simulink model "MATE_PMSMDynamicSwitches"  (R2024b)
settings: Solver=FixedStepDiscrete  StartTime=0.0  StopTime=0.6  RelTol=1e-3  AbsTol=1e-3
PostLoadFcn:
  | Ts = 2e-6;
  | PMSMDynamicSwitches_init
InitFcn:
  | Ts = 2e-6;
  | PMSMDynamicSwitches_init
values from neighbouring files (symbols this model uses):
  J = 0.2    [PMSMDynamicSwitches_init.m]
  Tmax = 1.5*N*PM*Imax    (= 27)    [PMSMDynamicSwitches_init.m]
  Tsc = 1/fc    (= 5e-05)    [PMSMDynamicSwitches_init.m]
libraries: fl_lib x24, nesl_utility x19, simulink x3, ee_lib x3, batteryecm_lib x1, eePmsmFieldOrientedControl x1
(part 2 of 2)

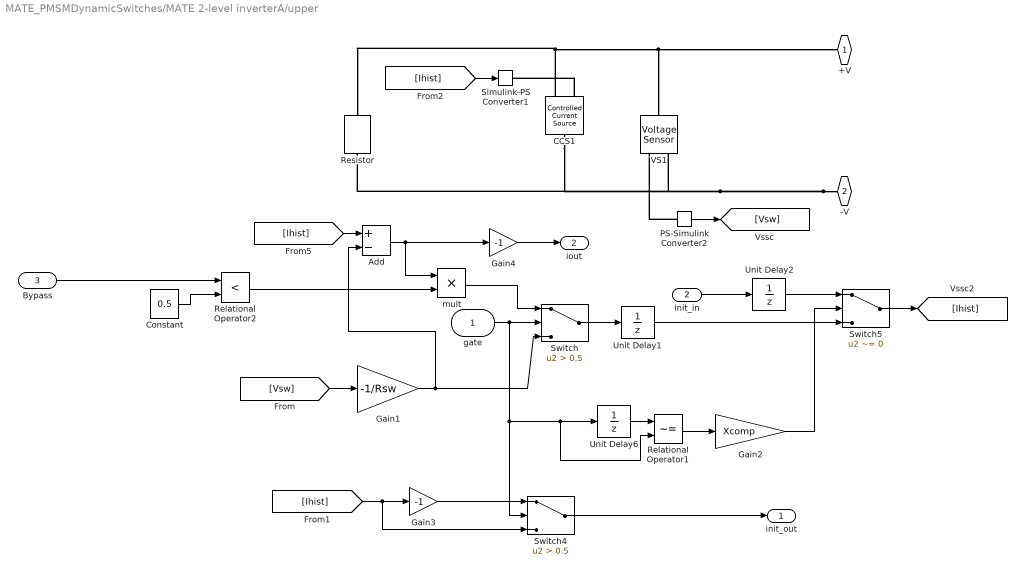
== system MATE_PMSMDynamicSwitches/MATE 2-level inverterA/upper ==
  gate : Inport
  init_in : Inport  Port=2
  Bypass : Inport  Port=3
  Add : Sum  Inputs=+-
  CCS1 : fl_lib/Electrical/Electrical Sources/Controlled Current Source
  Constant : Constant  Value=0.5
  Gain1 : Gain  Gain=-1/Rsw
  Gain2 : Gain  Gain=Xcomp
  Gain3 : Gain  Gain=-1
  Gain4 : Gain  Gain=-1
  PS-Simulink Converter2 : nesl_utility/PS-Simulink Converter  PhysicalDomain=network_engine_domain  SubClassName=ps_output  LeftPortType=input  RightPortType=output  PseudoPeriodic=off  Frequencies=[]  VectorFormat=inherit  Unit=inherit  AffineConversion=off
  Relational Operator1 : RelationalOperator  Operator=~=  OutDataTypeStr=boolean  RndMeth=Simplest  InputSameDT=off
  Relational Operator2 : RelationalOperator  Operator=<  OutDataTypeStr=boolean  RndMeth=Simplest  InputSameDT=off
  Resistor : fl_lib/Electrical/Electrical Elements/Resistor  R=Rsw Ohm  i_specify=off  i_priority=None  i=0 A  i_nominal_specify=off  i_nominal_value=1  i_nominal_unit=A  v_specify=off  v_priority=None  v=0 V  v_nominal_specify=off  v_nominal_value=1  v_nominal_unit=V
  Simulink-PS Converter1 : nesl_utility/Simulink-PS Converter  PhysicalDomain=network_engine_domain  SubClassName=ps_input  LeftPortType=input  RightPortType=output  PseudoPeriodic=off  Frequencies=[]  NoiseDistribution=none  NoiseParameters=[]  Unit=1  AffineConversion=off  FilteringAndDerivatives=provide  SimscapeFilterOrder=1  InputFilterTimeConstant=0.001  UdotUserProvided=0
  Switch : Switch  Criteria=u2 > Threshold  Threshold=0.5  SaturateOnIntegerOverflow=off  InputSameDT=off
  Switch4 : Switch  Criteria=u2 > Threshold  Threshold=0.5  SaturateOnIntegerOverflow=off  InputSameDT=off
  Switch5 : Switch  Criteria=u2 ~= 0  Threshold=0.5  SaturateOnIntegerOverflow=off  InputSameDT=off
  Unit Delay1 : UnitDelay  SampleTime=-1  HasFrameUpgradeWarning=on
  Unit Delay2 : UnitDelay  SampleTime=Ts  HasFrameUpgradeWarning=on
  Unit Delay6 : UnitDelay  SampleTime=Ts  HasFrameUpgradeWarning=on
  VS1 : fl_lib/Electrical/Electrical Sensors/Voltage Sensor
  mult : Product
  +V : PMIOPort  Side=Left
  -V : PMIOPort  Port=2  Side=Right
  init_out : Outport
  iout : Outport  Port=2
  wires:
  Constant/1 -> Relational Operator2/2
  Unit Delay2/1 -> Switch5/1
  [Ihist] -> Gain3/1, Switch4/3
  Relational Operator2/1 -> mult/2
  Bypass/1 -> Relational Operator2/1
  mult/1 -> Switch/1
  [Ihist] -> Simulink-PS Converter1/1
  Switch/1 -> Unit Delay1/1
  [Vsw] -> Gain1/1
  PS-Simulink Converter2/1 -> [Vsw]
  [Ihist] -> Add/1
  Gain1/1 -> Switch/3, Add/2
  Add/1 -> Gain4/1, mult/1
  Unit Delay1/1 -> Switch5/3
  Switch4/1 -> init_out/1
  Gain3/1 -> Switch4/1
  Gain2/1 -> Switch5/2
  Unit Delay6/1 -> Relational Operator1/1
  gate/1 -> Switch4/2, Unit Delay6/1, Relational Operator1/2, Switch/2
  Relational Operator1/1 -> Gain2/1
  init_in/1 -> Unit Delay2/1
  Switch5/1 -> [Ihist]
  Gain4/1 -> iout/1
  connections:
  CCS1/RConn2 -- +V/RConn1 -- VS1/LConn1 -- Resistor/LConn1
  CCS1/RConn1 -- Simulink-PS Converter1/RConn1
  PS-Simulink Converter2/LConn1 -- VS1/RConn1
  -V/RConn1 -- VS1/RConn2 -- CCS1/LConn1 -- Resistor/RConn1

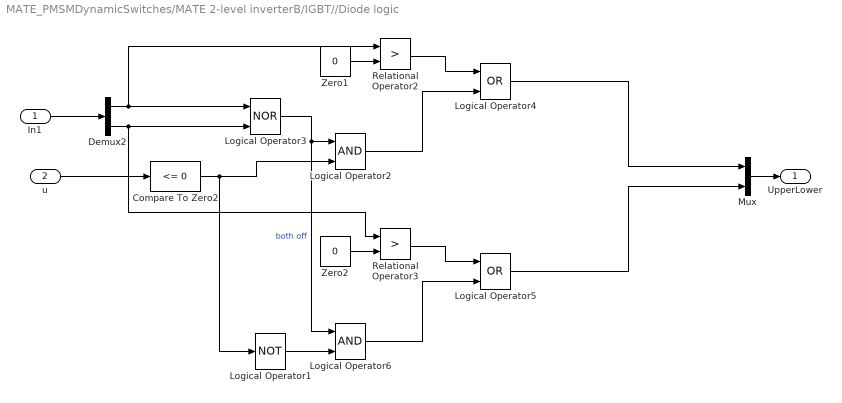
== system MATE_PMSMDynamicSwitches/MATE 2-level inverterB/IGBT//Diode logic ==
  In1 : Inport
  u : Inport  Port=2
  Compare To Zero2 : simulink/Logic and Bit Operations/Compare To Zero  relop=<=  OutDataTypeStr=uint8
  Demux2 : Demux  Outputs=2
  Logical Operator1 : Logic  Operator=NOT  AllPortsSameDT=off  OutDataTypeStr=boolean
  Logical Operator2 : Logic  AllPortsSameDT=off  OutDataTypeStr=boolean
  Logical Operator3 : Logic  Operator=NOR  AllPortsSameDT=off  OutDataTypeStr=boolean
  Logical Operator4 : Logic  Operator=OR  AllPortsSameDT=off  OutDataTypeStr=boolean
  Logical Operator5 : Logic  Operator=OR  AllPortsSameDT=off  OutDataTypeStr=boolean
  Logical Operator6 : Logic  AllPortsSameDT=off  OutDataTypeStr=boolean
  Mux : Mux  Inputs=2
  Relational Operator2 : RelationalOperator  Operator=>  OutDataTypeStr=boolean  InputSameDT=off
  Relational Operator3 : RelationalOperator  Operator=>  OutDataTypeStr=boolean  InputSameDT=off
  Zero1 : Constant  Value=0  OutDataTypeStr=Inherit: Inherit via back propagation
  Zero2 : Constant  Value=0  OutDataTypeStr=Inherit: Inherit via back propagation
  UpperLower : Outport
  wires:
  Mux/1 -> UpperLower/1
  Logical Operator5/1 -> Mux/2
  Logical Operator4/1 -> Mux/1
  In1/1 -> Demux2/1
  u/1 -> Compare To Zero2/1
  Logical Operator1/1 -> Logical Operator6/2
  Relational Operator3/1 -> Logical Operator5/1
  Logical Operator2/1 -> Logical Operator4/2
  Zero2/1 -> Relational Operator3/2
  Demux2/2 -> Relational Operator3/1, Logical Operator3/2
  Logical Operator6/1 -> Logical Operator5/2
  Compare To Zero2/1 -> Logical Operator2/2, Logical Operator1/1
  Zero1/1 -> Relational Operator2/2
  Logical Operator3/1 -> Logical Operator2/1, Logical Operator6/1  "both off"
  Relational Operator2/1 -> Logical Operator4/1
  Demux2/1 -> Relational Operator2/1, Logical Operator3/1

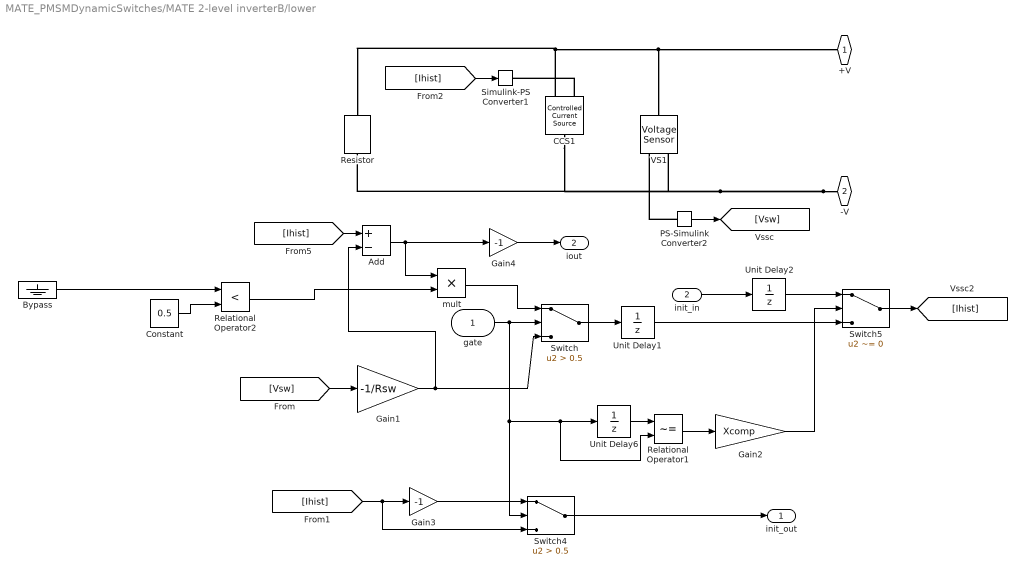
== system MATE_PMSMDynamicSwitches/MATE 2-level inverterB/lower ==
  gate : Inport
  init_in : Inport  Port=2
  Add : Sum  Inputs=+-
  Bypass : Ground
  CCS1 : fl_lib/Electrical/Electrical Sources/Controlled Current Source
  Constant : Constant  Value=0.5
  Gain1 : Gain  Gain=-1/Rsw
  Gain2 : Gain  Gain=Xcomp
  Gain3 : Gain  Gain=-1
  Gain4 : Gain  Gain=-1
  PS-Simulink Converter2 : nesl_utility/PS-Simulink Converter  PhysicalDomain=network_engine_domain  SubClassName=ps_output  LeftPortType=input  RightPortType=output  PseudoPeriodic=off  Frequencies=[]  VectorFormat=inherit  Unit=inherit  AffineConversion=off
  Relational Operator1 : RelationalOperator  Operator=~=  OutDataTypeStr=boolean  RndMeth=Simplest  InputSameDT=off
  Relational Operator2 : RelationalOperator  Operator=<  OutDataTypeStr=boolean  RndMeth=Simplest  InputSameDT=off
  Resistor : fl_lib/Electrical/Electrical Elements/Resistor  R=Rsw Ohm  i_specify=off  i_priority=None  i=0 A  i_nominal_specify=off  i_nominal_value=1  i_nominal_unit=A  v_specify=off  v_priority=None  v=0 V  v_nominal_specify=off  v_nominal_value=1  v_nominal_unit=V
  Simulink-PS Converter1 : nesl_utility/Simulink-PS Converter  PhysicalDomain=network_engine_domain  SubClassName=ps_input  LeftPortType=input  RightPortType=output  PseudoPeriodic=off  Frequencies=[]  NoiseDistribution=none  NoiseParameters=[]  Unit=1  AffineConversion=off  FilteringAndDerivatives=provide  SimscapeFilterOrder=1  InputFilterTimeConstant=0.001  UdotUserProvided=0
  Switch : Switch  Criteria=u2 > Threshold  Threshold=0.5  SaturateOnIntegerOverflow=off  InputSameDT=off
  Switch4 : Switch  Criteria=u2 > Threshold  Threshold=0.5  SaturateOnIntegerOverflow=off  InputSameDT=off
  Switch5 : Switch  Criteria=u2 ~= 0  Threshold=0.5  SaturateOnIntegerOverflow=off  InputSameDT=off
  Unit Delay1 : UnitDelay  SampleTime=-1  HasFrameUpgradeWarning=on
  Unit Delay2 : UnitDelay  SampleTime=Ts  HasFrameUpgradeWarning=on
  Unit Delay6 : UnitDelay  SampleTime=Ts  HasFrameUpgradeWarning=on
  VS1 : fl_lib/Electrical/Electrical Sensors/Voltage Sensor
  mult : Product
  +V : PMIOPort  Side=Left
  -V : PMIOPort  Port=2  Side=Right
  init_out : Outport
  iout : Outport  Port=2
  wires:
  Constant/1 -> Relational Operator2/2
  Unit Delay2/1 -> Switch5/1
  [Ihist] -> Gain3/1, Switch4/3
  Relational Operator2/1 -> mult/2
  Bypass/1 -> Relational Operator2/1
  mult/1 -> Switch/1
  [Ihist] -> Simulink-PS Converter1/1
  Switch/1 -> Unit Delay1/1
  [Vsw] -> Gain1/1
  PS-Simulink Converter2/1 -> [Vsw]
  [Ihist] -> Add/1
  Gain1/1 -> Switch/3, Add/2
  Add/1 -> Gain4/1, mult/1
  Unit Delay1/1 -> Switch5/3
  Switch4/1 -> init_out/1
  Gain3/1 -> Switch4/1
  Gain2/1 -> Switch5/2
  Unit Delay6/1 -> Relational Operator1/1
  gate/1 -> Switch4/2, Unit Delay6/1, Relational Operator1/2, Switch/2
  Relational Operator1/1 -> Gain2/1
  init_in/1 -> Unit Delay2/1
  Switch5/1 -> [Ihist]
  Gain4/1 -> iout/1
  connections:
  CCS1/RConn2 -- +V/RConn1 -- VS1/LConn1 -- Resistor/LConn1
  CCS1/RConn1 -- Simulink-PS Converter1/RConn1
  PS-Simulink Converter2/LConn1 -- VS1/RConn1
  -V/RConn1 -- VS1/RConn2 -- CCS1/LConn1 -- Resistor/RConn1

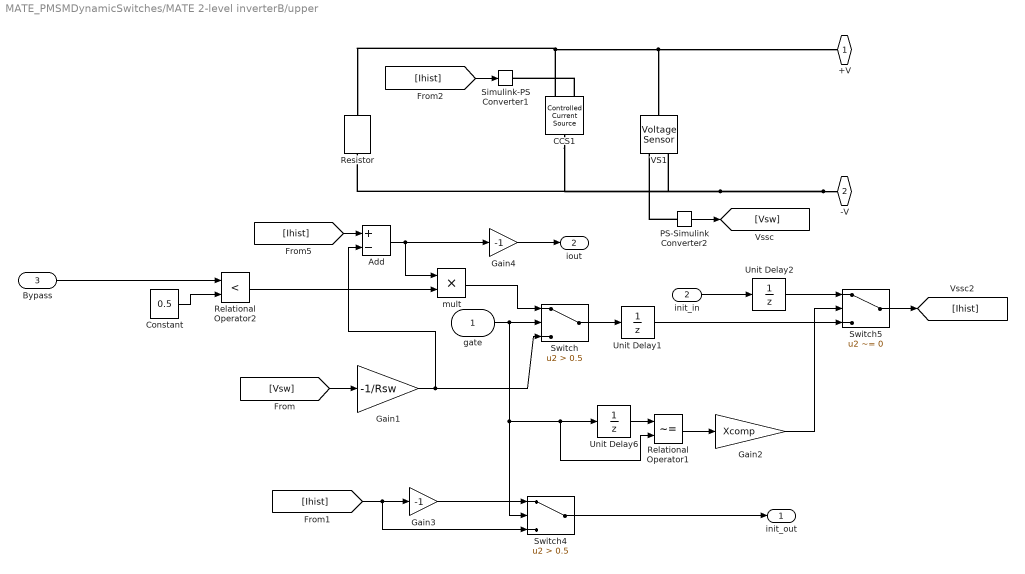
== system MATE_PMSMDynamicSwitches/MATE 2-level inverterB/upper ==
  gate : Inport
  init_in : Inport  Port=2
  Bypass : Inport  Port=3
  Add : Sum  Inputs=+-
  CCS1 : fl_lib/Electrical/Electrical Sources/Controlled Current Source
  Constant : Constant  Value=0.5
  Gain1 : Gain  Gain=-1/Rsw
  Gain2 : Gain  Gain=Xcomp
  Gain3 : Gain  Gain=-1
  Gain4 : Gain  Gain=-1
  PS-Simulink Converter2 : nesl_utility/PS-Simulink Converter  PhysicalDomain=network_engine_domain  SubClassName=ps_output  LeftPortType=input  RightPortType=output  PseudoPeriodic=off  Frequencies=[]  VectorFormat=inherit  Unit=inherit  AffineConversion=off
  Relational Operator1 : RelationalOperator  Operator=~=  OutDataTypeStr=boolean  RndMeth=Simplest  InputSameDT=off
  Relational Operator2 : RelationalOperator  Operator=<  OutDataTypeStr=boolean  RndMeth=Simplest  InputSameDT=off
  Resistor : fl_lib/Electrical/Electrical Elements/Resistor  R=Rsw Ohm  i_specify=off  i_priority=None  i=0 A  i_nominal_specify=off  i_nominal_value=1  i_nominal_unit=A  v_specify=off  v_priority=None  v=0 V  v_nominal_specify=off  v_nominal_value=1  v_nominal_unit=V
  Simulink-PS Converter1 : nesl_utility/Simulink-PS Converter  PhysicalDomain=network_engine_domain  SubClassName=ps_input  LeftPortType=input  RightPortType=output  PseudoPeriodic=off  Frequencies=[]  NoiseDistribution=none  NoiseParameters=[]  Unit=1  AffineConversion=off  FilteringAndDerivatives=provide  SimscapeFilterOrder=1  InputFilterTimeConstant=0.001  UdotUserProvided=0
  Switch : Switch  Criteria=u2 > Threshold  Threshold=0.5  SaturateOnIntegerOverflow=off  InputSameDT=off
  Switch4 : Switch  Criteria=u2 > Threshold  Threshold=0.5  SaturateOnIntegerOverflow=off  InputSameDT=off
  Switch5 : Switch  Criteria=u2 ~= 0  Threshold=0.5  SaturateOnIntegerOverflow=off  InputSameDT=off
  Unit Delay1 : UnitDelay  SampleTime=-1  HasFrameUpgradeWarning=on
  Unit Delay2 : UnitDelay  SampleTime=Ts  HasFrameUpgradeWarning=on
  Unit Delay6 : UnitDelay  SampleTime=Ts  HasFrameUpgradeWarning=on
  VS1 : fl_lib/Electrical/Electrical Sensors/Voltage Sensor
  mult : Product
  +V : PMIOPort  Side=Left
  -V : PMIOPort  Port=2  Side=Right
  init_out : Outport
  iout : Outport  Port=2
  wires:
  Constant/1 -> Relational Operator2/2
  Unit Delay2/1 -> Switch5/1
  [Ihist] -> Gain3/1, Switch4/3
  Relational Operator2/1 -> mult/2
  Bypass/1 -> Relational Operator2/1
  mult/1 -> Switch/1
  [Ihist] -> Simulink-PS Converter1/1
  Switch/1 -> Unit Delay1/1
  [Vsw] -> Gain1/1
  PS-Simulink Converter2/1 -> [Vsw]
  [Ihist] -> Add/1
  Gain1/1 -> Switch/3, Add/2
  Add/1 -> Gain4/1, mult/1
  Unit Delay1/1 -> Switch5/3
  Switch4/1 -> init_out/1
  Gain3/1 -> Switch4/1
  Gain2/1 -> Switch5/2
  Unit Delay6/1 -> Relational Operator1/1
  gate/1 -> Switch4/2, Unit Delay6/1, Relational Operator1/2, Switch/2
  Relational Operator1/1 -> Gain2/1
  init_in/1 -> Unit Delay2/1
  Switch5/1 -> [Ihist]
  Gain4/1 -> iout/1
  connections:
  CCS1/RConn2 -- +V/RConn1 -- VS1/LConn1 -- Resistor/LConn1
  CCS1/RConn1 -- Simulink-PS Converter1/RConn1
  PS-Simulink Converter2/LConn1 -- VS1/RConn1
  -V/RConn1 -- VS1/RConn2 -- CCS1/LConn1 -- Resistor/RConn1

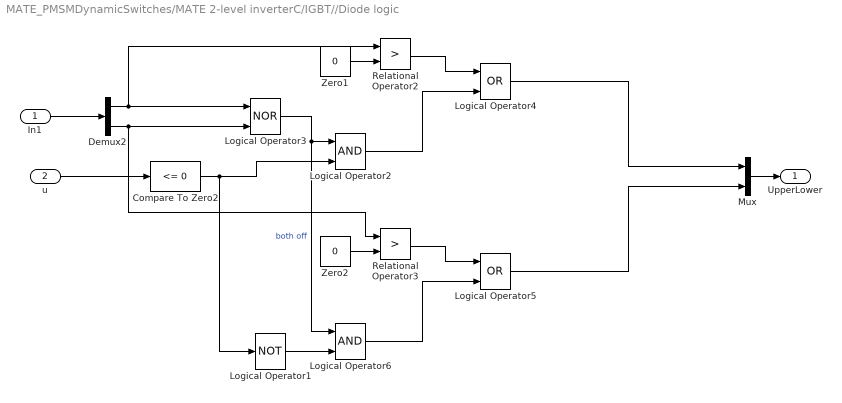
== system MATE_PMSMDynamicSwitches/MATE 2-level inverterC/IGBT//Diode logic ==
  In1 : Inport
  u : Inport  Port=2
  Compare To Zero2 : simulink/Logic and Bit Operations/Compare To Zero  relop=<=  OutDataTypeStr=uint8
  Demux2 : Demux  Outputs=2
  Logical Operator1 : Logic  Operator=NOT  AllPortsSameDT=off  OutDataTypeStr=boolean
  Logical Operator2 : Logic  AllPortsSameDT=off  OutDataTypeStr=boolean
  Logical Operator3 : Logic  Operator=NOR  AllPortsSameDT=off  OutDataTypeStr=boolean
  Logical Operator4 : Logic  Operator=OR  AllPortsSameDT=off  OutDataTypeStr=boolean
  Logical Operator5 : Logic  Operator=OR  AllPortsSameDT=off  OutDataTypeStr=boolean
  Logical Operator6 : Logic  AllPortsSameDT=off  OutDataTypeStr=boolean
  Mux : Mux  Inputs=2
  Relational Operator2 : RelationalOperator  Operator=>  OutDataTypeStr=boolean  InputSameDT=off
  Relational Operator3 : RelationalOperator  Operator=>  OutDataTypeStr=boolean  InputSameDT=off
  Zero1 : Constant  Value=0  OutDataTypeStr=Inherit: Inherit via back propagation
  Zero2 : Constant  Value=0  OutDataTypeStr=Inherit: Inherit via back propagation
  UpperLower : Outport
  wires:
  Mux/1 -> UpperLower/1
  Logical Operator5/1 -> Mux/2
  Logical Operator4/1 -> Mux/1
  In1/1 -> Demux2/1
  u/1 -> Compare To Zero2/1
  Logical Operator1/1 -> Logical Operator6/2
  Relational Operator3/1 -> Logical Operator5/1
  Logical Operator2/1 -> Logical Operator4/2
  Zero2/1 -> Relational Operator3/2
  Demux2/2 -> Relational Operator3/1, Logical Operator3/2
  Logical Operator6/1 -> Logical Operator5/2
  Compare To Zero2/1 -> Logical Operator2/2, Logical Operator1/1
  Zero1/1 -> Relational Operator2/2
  Logical Operator3/1 -> Logical Operator2/1, Logical Operator6/1  "both off"
  Relational Operator2/1 -> Logical Operator4/1
  Demux2/1 -> Relational Operator2/1, Logical Operator3/1

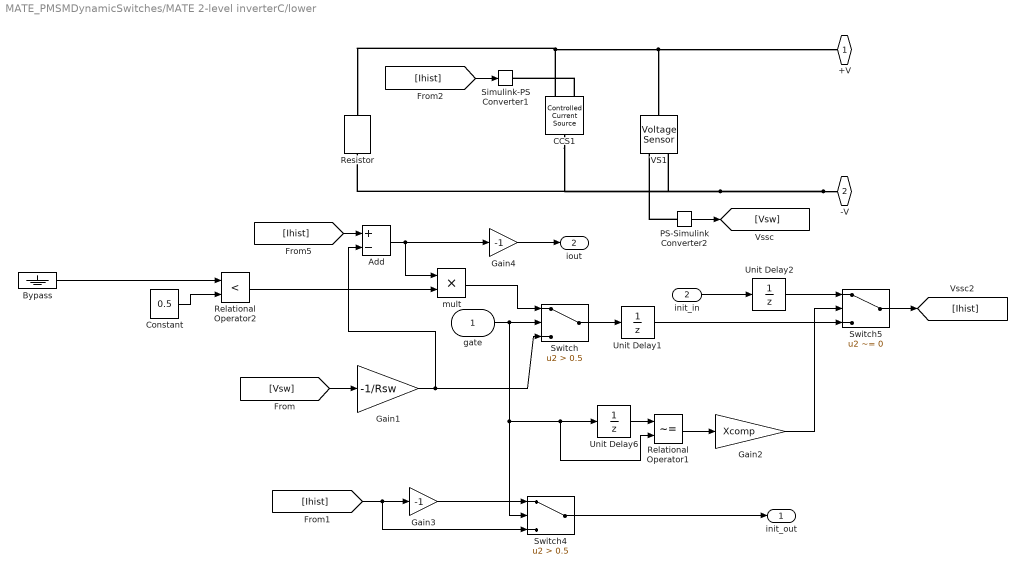
== system MATE_PMSMDynamicSwitches/MATE 2-level inverterC/lower ==
  gate : Inport
  init_in : Inport  Port=2
  Add : Sum  Inputs=+-
  Bypass : Ground
  CCS1 : fl_lib/Electrical/Electrical Sources/Controlled Current Source
  Constant : Constant  Value=0.5
  Gain1 : Gain  Gain=-1/Rsw
  Gain2 : Gain  Gain=Xcomp
  Gain3 : Gain  Gain=-1
  Gain4 : Gain  Gain=-1
  PS-Simulink Converter2 : nesl_utility/PS-Simulink Converter  PhysicalDomain=network_engine_domain  SubClassName=ps_output  LeftPortType=input  RightPortType=output  PseudoPeriodic=off  Frequencies=[]  VectorFormat=inherit  Unit=inherit  AffineConversion=off
  Relational Operator1 : RelationalOperator  Operator=~=  OutDataTypeStr=boolean  RndMeth=Simplest  InputSameDT=off
  Relational Operator2 : RelationalOperator  Operator=<  OutDataTypeStr=boolean  RndMeth=Simplest  InputSameDT=off
  Resistor : fl_lib/Electrical/Electrical Elements/Resistor  R=Rsw Ohm  i_specify=off  i_priority=None  i=0 A  i_nominal_specify=off  i_nominal_value=1  i_nominal_unit=A  v_specify=off  v_priority=None  v=0 V  v_nominal_specify=off  v_nominal_value=1  v_nominal_unit=V
  Simulink-PS Converter1 : nesl_utility/Simulink-PS Converter  PhysicalDomain=network_engine_domain  SubClassName=ps_input  LeftPortType=input  RightPortType=output  PseudoPeriodic=off  Frequencies=[]  NoiseDistribution=none  NoiseParameters=[]  Unit=1  AffineConversion=off  FilteringAndDerivatives=provide  SimscapeFilterOrder=1  InputFilterTimeConstant=0.001  UdotUserProvided=0
  Switch : Switch  Criteria=u2 > Threshold  Threshold=0.5  SaturateOnIntegerOverflow=off  InputSameDT=off
  Switch4 : Switch  Criteria=u2 > Threshold  Threshold=0.5  SaturateOnIntegerOverflow=off  InputSameDT=off
  Switch5 : Switch  Criteria=u2 ~= 0  Threshold=0.5  SaturateOnIntegerOverflow=off  InputSameDT=off
  Unit Delay1 : UnitDelay  SampleTime=-1  HasFrameUpgradeWarning=on
  Unit Delay2 : UnitDelay  SampleTime=Ts  HasFrameUpgradeWarning=on
  Unit Delay6 : UnitDelay  SampleTime=Ts  HasFrameUpgradeWarning=on
  VS1 : fl_lib/Electrical/Electrical Sensors/Voltage Sensor
  mult : Product
  +V : PMIOPort  Side=Left
  -V : PMIOPort  Port=2  Side=Right
  init_out : Outport
  iout : Outport  Port=2
  wires:
  Constant/1 -> Relational Operator2/2
  Unit Delay2/1 -> Switch5/1
  [Ihist] -> Gain3/1, Switch4/3
  Relational Operator2/1 -> mult/2
  Bypass/1 -> Relational Operator2/1
  mult/1 -> Switch/1
  [Ihist] -> Simulink-PS Converter1/1
  Switch/1 -> Unit Delay1/1
  [Vsw] -> Gain1/1
  PS-Simulink Converter2/1 -> [Vsw]
  [Ihist] -> Add/1
  Gain1/1 -> Switch/3, Add/2
  Add/1 -> Gain4/1, mult/1
  Unit Delay1/1 -> Switch5/3
  Switch4/1 -> init_out/1
  Gain3/1 -> Switch4/1
  Gain2/1 -> Switch5/2
  Unit Delay6/1 -> Relational Operator1/1
  gate/1 -> Switch4/2, Unit Delay6/1, Relational Operator1/2, Switch/2
  Relational Operator1/1 -> Gain2/1
  init_in/1 -> Unit Delay2/1
  Switch5/1 -> [Ihist]
  Gain4/1 -> iout/1
  connections:
  CCS1/RConn2 -- +V/RConn1 -- VS1/LConn1 -- Resistor/LConn1
  CCS1/RConn1 -- Simulink-PS Converter1/RConn1
  PS-Simulink Converter2/LConn1 -- VS1/RConn1
  -V/RConn1 -- VS1/RConn2 -- CCS1/LConn1 -- Resistor/RConn1

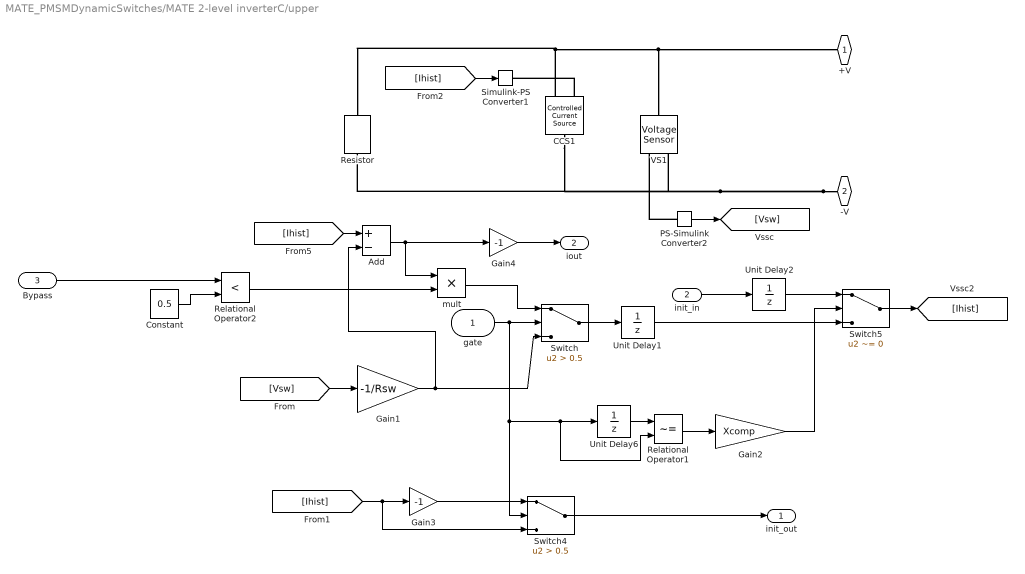
== system MATE_PMSMDynamicSwitches/MATE 2-level inverterC/upper ==
  gate : Inport
  init_in : Inport  Port=2
  Bypass : Inport  Port=3
  Add : Sum  Inputs=+-
  CCS1 : fl_lib/Electrical/Electrical Sources/Controlled Current Source
  Constant : Constant  Value=0.5
  Gain1 : Gain  Gain=-1/Rsw
  Gain2 : Gain  Gain=Xcomp
  Gain3 : Gain  Gain=-1
  Gain4 : Gain  Gain=-1
  PS-Simulink Converter2 : nesl_utility/PS-Simulink Converter  PhysicalDomain=network_engine_domain  SubClassName=ps_output  LeftPortType=input  RightPortType=output  PseudoPeriodic=off  Frequencies=[]  VectorFormat=inherit  Unit=inherit  AffineConversion=off
  Relational Operator1 : RelationalOperator  Operator=~=  OutDataTypeStr=boolean  RndMeth=Simplest  InputSameDT=off
  Relational Operator2 : RelationalOperator  Operator=<  OutDataTypeStr=boolean  RndMeth=Simplest  InputSameDT=off
  Resistor : fl_lib/Electrical/Electrical Elements/Resistor  R=Rsw Ohm  i_specify=off  i_priority=None  i=0 A  i_nominal_specify=off  i_nominal_value=1  i_nominal_unit=A  v_specify=off  v_priority=None  v=0 V  v_nominal_specify=off  v_nominal_value=1  v_nominal_unit=V
  Simulink-PS Converter1 : nesl_utility/Simulink-PS Converter  PhysicalDomain=network_engine_domain  SubClassName=ps_input  LeftPortType=input  RightPortType=output  PseudoPeriodic=off  Frequencies=[]  NoiseDistribution=none  NoiseParameters=[]  Unit=1  AffineConversion=off  FilteringAndDerivatives=provide  SimscapeFilterOrder=1  InputFilterTimeConstant=0.001  UdotUserProvided=0
  Switch : Switch  Criteria=u2 > Threshold  Threshold=0.5  SaturateOnIntegerOverflow=off  InputSameDT=off
  Switch4 : Switch  Criteria=u2 > Threshold  Threshold=0.5  SaturateOnIntegerOverflow=off  InputSameDT=off
  Switch5 : Switch  Criteria=u2 ~= 0  Threshold=0.5  SaturateOnIntegerOverflow=off  InputSameDT=off
  Unit Delay1 : UnitDelay  SampleTime=-1  HasFrameUpgradeWarning=on
  Unit Delay2 : UnitDelay  SampleTime=Ts  HasFrameUpgradeWarning=on
  Unit Delay6 : UnitDelay  SampleTime=Ts  HasFrameUpgradeWarning=on
  VS1 : fl_lib/Electrical/Electrical Sensors/Voltage Sensor
  mult : Product
  +V : PMIOPort  Side=Left
  -V : PMIOPort  Port=2  Side=Right
  init_out : Outport
  iout : Outport  Port=2
  wires:
  Constant/1 -> Relational Operator2/2
  Unit Delay2/1 -> Switch5/1
  [Ihist] -> Gain3/1, Switch4/3
  Relational Operator2/1 -> mult/2
  Bypass/1 -> Relational Operator2/1
  mult/1 -> Switch/1
  [Ihist] -> Simulink-PS Converter1/1
  Switch/1 -> Unit Delay1/1
  [Vsw] -> Gain1/1
  PS-Simulink Converter2/1 -> [Vsw]
  [Ihist] -> Add/1
  Gain1/1 -> Switch/3, Add/2
  Add/1 -> Gain4/1, mult/1
  Unit Delay1/1 -> Switch5/3
  Switch4/1 -> init_out/1
  Gain3/1 -> Switch4/1
  Gain2/1 -> Switch5/2
  Unit Delay6/1 -> Relational Operator1/1
  gate/1 -> Switch4/2, Unit Delay6/1, Relational Operator1/2, Switch/2
  Relational Operator1/1 -> Gain2/1
  init_in/1 -> Unit Delay2/1
  Switch5/1 -> [Ihist]
  Gain4/1 -> iout/1
  connections:
  CCS1/RConn2 -- +V/RConn1 -- VS1/LConn1 -- Resistor/LConn1
  CCS1/RConn1 -- Simulink-PS Converter1/RConn1
  PS-Simulink Converter2/LConn1 -- VS1/RConn1
  -V/RConn1 -- VS1/RConn2 -- CCS1/LConn1 -- Resistor/RConn1
